simulink model "Adaptive_Controller_Example"  (R2013b)
settings: Solver=ode3  StartTime=0.0  StopTime=50  FixedStep=0.0001  RelTol=1e-3
PreLoadFcn:
  | R= 2.0; % Ohms
  | L= 0.5; % Henrys
  | Km = .015; % torque constant
  | Kb = .015; % emf constant
  | B = 0.2; % Nms
  | J= 0.02; % kg.m^2
  | Kc= 1;
  | Kf = 0.2;
  | gamma = 0.1;
libraries: simulink x2
settings Model: Creator=cpatel  LastModifiedBy=cpatel
settings OptimizationCC: ExpressionDepthLimit=2147483647
settings DebuggingCC: StateNameClashWarn=warning
settings GRTTargetCC: CombineOutputUpdateFcns=off  GRTInterface=on

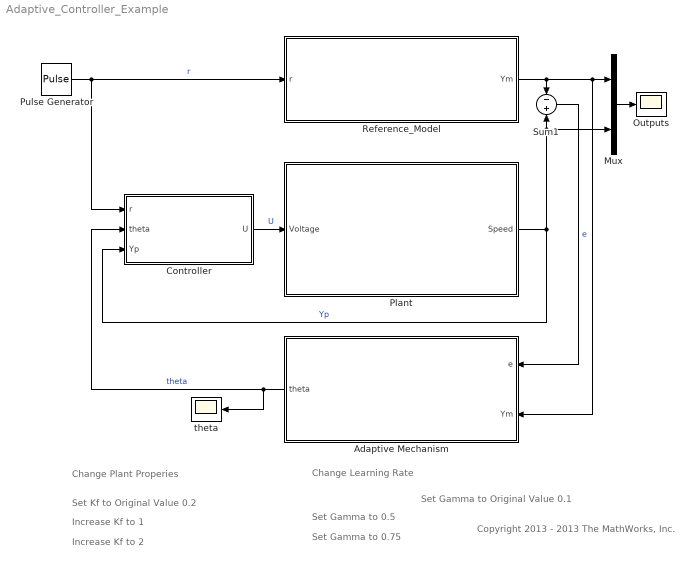
== system Adaptive_Controller_Example ==
  note: Copyright 2013 - 2013 The MathWorks, Inc.
  note: Change Learning Rate
  note: Change Plant Properies
  note: Increase Kf to 1
  note: Set Kf to Original Value 0.2
  note: Increase Kf to 2
  note: Set Gamma to 0.5
  note: Set Gamma to Original Value 0.1
  note: Set Gamma to 0.75
  Adaptive Mechanism : Subsystem
  Controller : Subsystem
  Mux : Mux  Inputs=2
  Outputs : Scope
      settings: ShowLegends=on  TimeRange=50  YMin=-0.25  YMax=3.25
  Plant : Subsystem
  Pulse Generator : DiscretePulseGenerator  PulseType=Time based  Amplitude=3.14  Period=10  PulseWidth=50
  Reference_Model : Subsystem
  Sum1 : Sum  Inputs=-|+
  theta : Scope
      settings: ShowLegends=on  TimeRange=50  YMin=1  YMax=4
  wires:
  Pulse Generator/1 -> Controller/1(r), Reference_Model/1(r)  "r"
  Plant/1(Speed) -> Controller/3(Yp), Sum1/2, Mux/2  "Yp"
  Mux/1 -> Outputs/1
  Adaptive Mechanism/1(theta) -> Controller/2(theta), theta/1  "theta"
  Sum1/1 -> Adaptive Mechanism/1(e)  "e"
  Controller/1(U) -> Plant/1(Voltage)  "U"
  Reference_Model/1(Ym) -> Sum1/1, Adaptive Mechanism/2(Ym), Mux/1

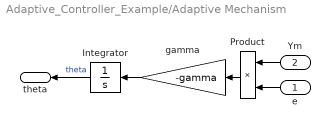
== system Adaptive_Controller_Example/Adaptive Mechanism ==
  e : Inport
  Ym : Inport  Port=2
  Integrator : Integrator  InitialCondition=1
  Product : Product
  gamma : Gain  Gain=-gamma
  theta : Outport
  wires:
  Integrator/1 -> theta/1  "theta"
  gamma/1 -> Integrator/1
  Product/1 -> gamma/1
  Ym/1 -> Product/1
  e/1 -> Product/2

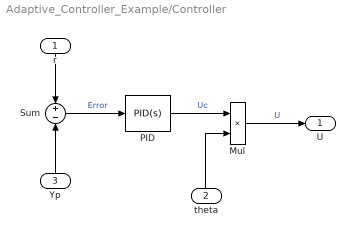
== system Adaptive_Controller_Example/Controller ==
  r : Inport
  theta : Inport  Port=2
  Yp : Inport  Port=3
  Mul : Product
  PID : simulink/Continuous/PID Controller  Controller=PID  TimeDomain=Continuous-time  SampleTime=1  IntegratorMethod=Forward Euler  FilterMethod=Forward Euler  Form=Parallel  P=30  I=100  D=0  N=100  InitialConditionSource=internal  InitialConditionForIntegrator=0  InitialConditionForFilter=0  ExternalReset=none  LimitOutput=off  UpperSaturationLimit=inf  LowerSaturationLimit=-inf  LinearizeAsGain=on  AntiWindupMode=none  Kb=1  TrackingMode=off  Kt=1  PParamMin=[]  PParamMax=[]  IParamMin=[]  IParamMax=[]  DParamMin=[]  DParamMax=[]  NParamMin=[]  NParamMax=[]  KbParamMin=[]  KbParamMax=[]  KtParamMin=[]  KtParamMax=[]  POutMin=[]  POutMax=[]  IOutMin=[]  IOutMax=[]  DOutMin=[]  DOutMax=[]  NOutMin=[]  NOutMax=[]  KbOutMin=[]  KbOutMax=[]  KtOutMin=[]  KtOutMax=[]  IntegratorOutMin=[]  IntegratorOutMax=[]  FilterOutMin=[]  FilterOutMax=[]  SumOutMin=[]  SumOutMax=[]  SumI1OutMin=[]  SumI1OutMax=[]  SumI2OutMin=[]  SumI2OutMax=[]  SumI3OutMin=[]  SumI3OutMax=[]  SumDOutMin=[]  SumDOutMax=[]  SaturationOutMin=[]  SaturationOutMax=[]  IntegratorContinuousStateAttributes=''  IntegratorStateMustResolveToSignalObject=off  IntegratorRTWStateStorageClass=Auto  FilterContinuousStateAttributes=''  FilterStateMustResolveToSignalObject=off  FilterRTWStateStorageClass=Auto
  Sum : Sum  Inputs=+|-
  U : Outport
  wires:
  theta/1 -> Mul/2
  r/1 -> Sum/1
  Yp/1 -> Sum/2
  PID/1 -> Mul/1  "Uc"
  Sum/1 -> PID/1  "Error"
  Mul/1 -> U/1  "U"

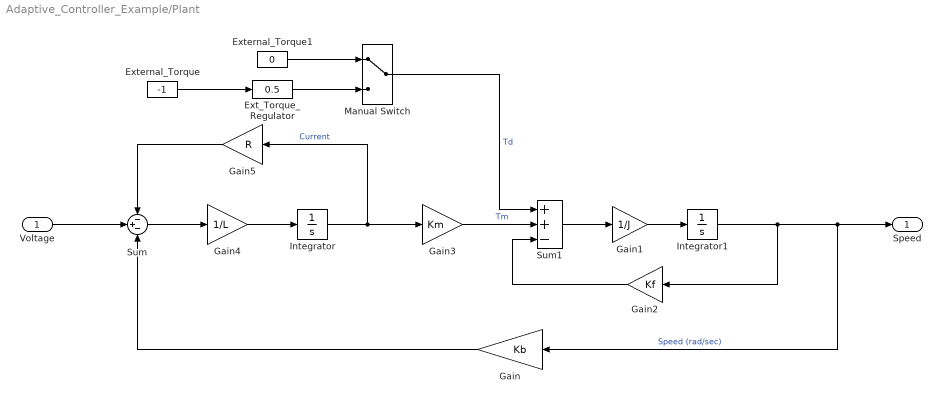
== system Adaptive_Controller_Example/Plant ==
  Voltage : Inport
  Ext_Torque_Regulator : simulink/Math Operations/Slider Gain  low=0  gain=0.5  high=1
  External_Torque : Constant  Value=-1
  External_Torque1 : Constant  Value=0
  Gain : Gain  Gain=Kb
  Gain1 : Gain  Gain=1/J
  Gain2 : Gain  Gain=Kf
  Gain3 : Gain  Gain=Km
  Gain4 : Gain  Gain=1/L
  Gain5 : Gain  Gain=R
  Integrator : Integrator  ContinuousStateAttributes='Current'
  Integrator1 : Integrator  ContinuousStateAttributes='Speed'
  Manual Switch : ManualSwitch
  Sum : Sum  Inputs=-+-
  Sum1 : Sum  Inputs=++-
  Speed : Outport
  wires:
  Sum/1 -> Gain4/1
  Gain3/1 -> Sum1/2  "Tm"
  Sum1/1 -> Gain1/1
  Integrator1/1 -> Gain/1, Speed/1, Gain2/1  "Speed (rad/sec)"
  Gain1/1 -> Integrator1/1
  Gain2/1 -> Sum1/3
  Integrator/1 -> Gain3/1, Gain5/1  "Current"
  Gain4/1 -> Integrator/1
  Gain/1 -> Sum/3
  Voltage/1 -> Sum/2
  Gain5/1 -> Sum/1
  Manual Switch/1 -> Sum1/1  "Td"
  External_Torque/1 -> Ext_Torque_Regulator/1
  External_Torque1/1 -> Manual Switch/1
  Ext_Torque_Regulator/1 -> Manual Switch/2

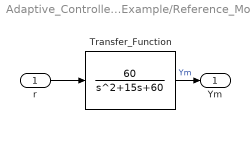
== system Adaptive_Controller_Example/Reference_Model ==
  r : Inport
  Transfer_Function : TransferFcn  Numerator=[60]  Denominator=[1 15 60]
  Ym : Outport
  wires:
  Transfer_Function/1 -> Ym/1  "Ym"
  r/1 -> Transfer_Function/1
